simulink library "motohawk_engine_lib"  (Simulink 6.3)
undefined symbols (not defined in the file or in its folder): cast_val, IndPowerMax, InjSequence, lookup_group, MAF_Sensor_p, motohawk_tex, motohawk_vardec_config_group, motohawk_vardec_path, SampleTime, SparkSequence, SteadyStateECT, txtTitle, WarmUpTimeConst
libraries: MotoHawk_lib x234, motohawk_annotations_lib x22, motohawk_control_primitives_lib x20, motohawk_engine_lib x8, motohawk_control_primitives_lib_new x3
(part 6 of 7)

== system motohawk_engine_lib/Closed-Loop O2 Control - Single Bank/O2 Control State Determination ==
  note: Desired equivalence ratio is within a delta of 1.0 (stoichiometric)
  note: Engine indicated work is above a threshold.
      | Usually a few minutes of idle time, to allow sensor warm-up.
  note: There are no O2 sensor faults
  note: Closed-loop O2 control is disabled when running
      | enrichment or engine in ransient
  O2ControlEnable [bool] : Inport
  DesEquivRatio : Inport  Port=2
  IndWork [kJ] : Inport  Port=3
  O2 Sensor Fault : Inport  Port=4
  Constant : Constant  OutDataTypeMode=single
  Logical Operator : Logic  AllPortsSameDT=off
  Logical Operator1 : Logic  Inputs=5
  Logical Operator3 : Logic  Operator=NOT  Inputs=3
  Relational Operator : RelationalOperator  Operator=<=  ZeroCross=off  InputSameDT=on
  Relational Operator1 : RelationalOperator  ZeroCross=off  InputSameDT=on
  Relational Operator2 : RelationalOperator  ZeroCross=off  InputSameDT=on
  Sum : Sum  Inputs=|++  SaturateOnIntegerOverflow=on
  Sum1 : Sum  Inputs=+-|  SaturateOnIntegerOverflow=on
  motohawk_TitleBlock : motohawk_annotations_lib/motohawk_TitleBlock  BlockType_='Mototron_Title_Block'  ttl=[txtTitle '\newline\rmClosed-Loop O2 Control State Determination']  copyright="'THE INFORMATION CONTAINED IN THIS\\newlineDRAWING IS THE SOLE PROPERTY OF\\newlineMOTOTRON.  ANY REPRODUCTION IN\\newline PART OR AS A WHOLE WITHOUT THE\\newlineWRITTEN PERMISSION OF MOTOTRON\\newline IS PROHIBITED.\\fontsize{16}\\rm\\copyright\\rm\\fontsize{10} 2005'"  address='\fontsize{22}\it\fontname{Arial Black}MotoTron Corporation \fontname{Arial}\fontsize{10}\newline505 Marion Road, Oshkosh, WI, 54901\newlinewww.mototron.com (734) 822-7700'  image_file='mh.jpg'  pretty_print=on  edit_text=[motohawk_tex(get_param(bdroot, 'Description')) '\rm\newline' motohawk_tex(get_param(gcs, 'Name'))]  edit_as=6
  motohawk_calibration : MotoHawk_lib/Calibration & Probing Blocks/motohawk_calibration  nam='O2ReadyIndWork'  val=O2ReadyIndWork  storage=Calibration  show_more=on  name_source=Use Parameter  data_type=Inherit from 'Default Value'  read_level=1  write_level=1  ovr_cals=on  view_as=Number  enum_struct={'Disabled', 'Enabled'}  vector_style=Wide Row  use_help_units=on  help='Minimum indicated work from engine before closed-loop O2 control will be enabled'  units='kJ'  use_header_enum=off  row_header_enum={}  col_header_enum={}  use_min_max=on  min_val=0  max_val=inf  use_precision=off  precision=''  gain=1  offset=0  exp=1  use_mototune_group=on  mototune_group='Engine Control | Run | O2 Control | O2 Control Config'
  motohawk_calibration1 : MotoHawk_lib/Calibration & Probing Blocks/motohawk_calibration  nam='O2EquivRatioDelta'  val=O2EquivRatioDelta  storage=Calibration  show_more=on  name_source=Use Parameter  data_type=Inherit from 'Default Value'  read_level=1  write_level=1  ovr_cals=on  view_as=Number  enum_struct={'Disabled', 'Enabled'}  vector_style=Wide Row  use_help_units=on  help='Equivalence ratio must be within this delta of stoichiometric to allow closed-loop O2 control'  units='ratio'  use_header_enum=off  row_header_enum={}  col_header_enum={}  use_min_max=on  min_val=0  max_val=1.0  use_precision=off  precision=''  gain=1  offset=0  exp=1  use_mototune_group=on  mototune_group='Engine Control | Run | O2 Control | O2 Control Config'
  motohawk_calibration2 : MotoHawk_lib/Calibration & Probing Blocks/motohawk_calibration  nam='O2ControlEnable'  val=O2ControlEnable  storage=Calibration  show_more=on  name_source=Use Parameter  data_type=boolean  read_level=1  write_level=1  ovr_cals=on  view_as=Enumeration  enum_struct={'Disabled', 'Enabled'}  vector_style=Wide Row  use_help_units=on  help='When enabled, the closed-loop O2 control algorithm is used'  units=''  use_header_enum=off  row_header_enum={}  col_header_enum={}  use_min_max=off  min_val=-inf  max_val=inf  use_precision=off  precision=''  gain=1  offset=0  exp=1  use_mototune_group=on  mototune_group='Engine Control | Run | O2 Control | O2 Control Config'
  motohawk_probe : MotoHawk_lib/Calibration & Probing Blocks/motohawk_probe  nam='O2Control'  show_more=on  name_source=Use Parameter  read_level=1  view_as=Enumeration  enum_struct={'Open-Loop', 'Closed-Loop'}  vector_style=Wide Row  use_help_units=on  help='Indicates whether closed-loop O2 control is currently enabled'  units=''  use_header_enum=off  row_header_enum={}  col_header_enum={}  use_precision=off  precision=''  gain=1  offset=0  exp=1  use_mototune_group=on  mototune_group='Engine Control | Run | O2 Control'
  O2Control : Outport
  wires:
  Logical Operator3/1 -> Logical Operator1/4
  O2 Sensor Fault/1 -> Logical Operator3/1
  Logical Operator/1 -> Logical Operator1/3
  Relational Operator2/1 -> Logical Operator1/2
  motohawk_calibration/1 -> Relational Operator2/2
  IndWork [kJ]/1 -> Relational Operator2/1
  Relational Operator1/1 -> Logical Operator/2
  Relational Operator/1 -> Logical Operator/1
  Sum1/1 -> Relational Operator1/2
  Sum/1 -> Relational Operator/2
  DesEquivRatio/1 -> Relational Operator/1, Relational Operator1/1
  Constant/1 -> Sum1/1, Sum/2
  motohawk_calibration1/1 -> Sum1/2, Sum/1
  Logical Operator1/1 -> O2Control/1, motohawk_probe/1
  O2ControlEnable [bool]/1 -> Logical Operator1/1
  motohawk_calibration2/1 -> Logical Operator1/5

== system motohawk_engine_lib/Crank Synchronous SIgnal/Once at Startup ==
  note: Sample Signal Once at Startup
  Signal_Time : Inport
  f : TriggerPort  TriggerType=function-call
  Signal_StartUp : Outport
  wires:
  Signal_Time/1 -> Signal_StartUp/1

== system motohawk_engine_lib/Crank Synchronous SIgnal/TDC and MID_TDC ==
  note: Average of Signal on TDC and MID_TDC
  Signal_Time : Inport
  f : TriggerPort  TriggerType=function-call
  Gain : Gain  Gain=1/2  SaturateOnIntegerOverflow=on
  Sum : Sum  Inputs=|++  InputSameDT=on
  Unit Delay : UnitDelay  SampleTime=-1
  Signal_Ave : Outport
  wires:
  Signal_Time/1 -> Sum/1, Unit Delay/1
  Gain/1 -> Signal_Ave/1
  Sum/1 -> Gain/1
  Unit Delay/1 -> Sum/2

== system motohawk_engine_lib/Idle Governor/Idle State Determination ==
  note: Idle States
      | 1 - Flaring
      | 2 - OnIdle
      | 3 - OffIdle
  RPM : Inport
  TargetRPM : Inport  Port=2
  ThrPos [%] : Inport  Port=3
  Determine if RPM is Falling : Subsystem
  Idle State Machine : Stateflow chart
  OnIdle State : motohawk_control_primitives_lib/CompareTo  op===  val=2
  Relational Operator : RelationalOperator  Operator=<  ZeroCross=off  InputSameDT=on
  Relational Operator1 : RelationalOperator  Operator=<  ZeroCross=off  InputSameDT=on
  Relational Operator2 : RelationalOperator  ZeroCross=off  InputSameDT=on
  Sum : Sum  Inputs=|++  SaturateOnIntegerOverflow=on  InputSameDT=on
  motohawk_TitleBlock : motohawk_annotations_lib/motohawk_TitleBlock  BlockType_='Mototron_Title_Block'  ttl='Idle Governor State Determination'  copyright="'THE INFORMATION CONTAINED IN THIS\\newlineDRAWING IS THE SOLE PROPERTY OF\\newlineMOTOTRON.  ANY REPRODUCTION IN\\newline PART OR AS A WHOLE WITHOUT THE\\newlineWRITTEN PERMISSION OF MOTOTRON\\newline IS PROHIBITED.\\fontsize{16}\\rm\\copyright\\rm\\fontsize{10} 2005'"  address='\fontsize{22}\it\fontname{Arial Black}MotoTron Corporation \fontname{Arial}\fontsize{10}\newline505 Marion Road, Oshkosh, WI, 54901\newlinewww.mototron.com (734) 822-7700'  image_file='mh.jpg'  pretty_print=on  edit_text=[motohawk_tex(get_param(bdroot, 'Description')) '\rm\newline' motohawk_tex(get_param(gcs, 'Name'))]  edit_as=6
  motohawk_calibration1 : MotoHawk_lib/Calibration & Probing Blocks/motohawk_calibration  nam='IdleEntryRPMDelta'  val=200  storage=Calibration  show_more=on  name_source=Use Parameter  data_type=Inherit from 'Default Value'  read_level=1  write_level=1  ovr_cals=on  view_as=Number  enum_struct={'Disabled', 'Enabled'}  vector_style=Wide Row  use_help_units=on  help='RPM must be within this delta from IdleTargetRPM to enter the Idle governor'  units='RPM'  use_header_enum=off  row_header_enum={}  col_header_enum={}  use_min_max=off  min_val=-inf  max_val=inf  use_precision=off  precision=''  gain=1  offset=0  exp=1  use_mototune_group=off  mototune_group=motohawk_vardec_path(gcb)
  motohawk_calibration3 : MotoHawk_lib/Calibration & Probing Blocks/motohawk_calibration  nam='IdleEntryThrPosThresh'  val=10  storage=Calibration  show_more=on  name_source=Use Parameter  data_type=Inherit from 'Default Value'  read_level=1  write_level=1  ovr_cals=on  view_as=Number  enum_struct={'Disabled', 'Enabled'}  vector_style=Wide Row  use_help_units=on  help='The throttle position must be closed below this threshold to enter the Idle governor'  units='%'  use_header_enum=off  row_header_enum={}  col_header_enum={}  use_min_max=off  min_val=-inf  max_val=inf  use_precision=off  precision=''  gain=1  offset=0  exp=1  use_mototune_group=off  mototune_group=motohawk_vardec_path(gcb)
  motohawk_calibration4 : MotoHawk_lib/Calibration & Probing Blocks/motohawk_calibration  nam='IdleExitThrPosThresh'  val=15  storage=Calibration  show_more=on  name_source=Use Parameter  data_type=Inherit from 'Default Value'  read_level=1  write_level=1  ovr_cals=on  view_as=Number  enum_struct={'Disabled', 'Enabled'}  vector_style=Wide Row  use_help_units=on  help='The throttle position must be opened above this threshold to exit the Idle governor'  units='%'  use_header_enum=off  row_header_enum={}  col_header_enum={}  use_min_max=off  min_val=-inf  max_val=inf  use_precision=off  precision=''  gain=1  offset=0  exp=1  use_mototune_group=off  mototune_group=motohawk_vardec_path(gcb)
  motohawk_calibration6 : MotoHawk_lib/Calibration & Probing Blocks/motohawk_calibration  nam='IdleEnable'  val=true  storage=Display  show_more=on  name_source=Use Parameter  data_type=Inherit from 'Default Value'  read_level=1  write_level=1  ovr_cals=on  view_as=Number  enum_struct={'Disabled', 'Enabled'}  vector_style=Wide Row  use_help_units=on  help='Allows the Idle governor to be manually enabled and disabled'  units='bool'  use_header_enum=off  row_header_enum={}  col_header_enum={}  use_min_max=off  min_val=-inf  max_val=inf  use_precision=off  precision=''  gain=1  offset=0  exp=1  use_mototune_group=off  mototune_group=motohawk_vardec_path(gcb)
  motohawk_probe1 : MotoHawk_lib/Calibration & Probing Blocks/motohawk_probe  nam='IdleState'  show_more=on  name_source=Use Parameter  read_level=1  view_as=Number  enum_struct={'Disabled', 'Enabled'}  vector_style=Wide Row  use_help_units=on  help="'0 - Off Idle    1 - On Idle'"  units=''  use_header_enum=off  row_header_enum={}  col_header_enum={}  use_precision=off  precision=''  gain=1  offset=0  exp=1  use_mototune_group=off  mototune_group=motohawk_vardec_path(gcb)
  OnIdle : Outport
  wires:
  Relational Operator1/1 -> Idle State Machine/4(ThrPosLow)
  Relational Operator/1 -> Idle State Machine/3(RPMLow)
  OnIdle State/1 -> OnIdle/1
  Idle State Machine/1(IdleState) -> OnIdle State/1, motohawk_probe1/1
  motohawk_calibration6/1 -> Idle State Machine/1(IdleEnable)
  Relational Operator2/1 -> Idle State Machine/5(ThrPosHigh)
  motohawk_calibration4/1 -> Relational Operator2/2
  motohawk_calibration3/1 -> Relational Operator1/2
  Sum/1 -> Relational Operator/2
  motohawk_calibration1/1 -> Sum/1
  TargetRPM/1 -> Sum/2
  Determine if RPM is Falling/1(RPM Falling) -> Idle State Machine/2(RPMFalling)
  RPM/1 -> Determine if RPM is Falling/1(RPM), Relational Operator/1
  ThrPos [%]/1 -> Relational Operator2/1, Relational Operator1/1

== system motohawk_engine_lib/Idle Governor/Ramp RPM ==
  note: y[k] = a*x[k] + (1-a)*y[k-1]
  note: where a = t/T
  OnIdle : Inport
  RPM : Inport  Port=2
  TargetRPM : Inport  Port=3
  Constant : Constant
  Logical Operator : Logic  Operator=NOT
  Preload lowpass filter with current RPM while not on Idle : Switch  Threshold=1  ZeroCross=off  SaturateOnIntegerOverflow=on  InputSameDT=on
  Product1 : Product  Inputs=*/  SaturateOnIntegerOverflow=on  InputSameDT=on
  Product2 : Product  SaturateOnIntegerOverflow=on  InputSameDT=on
  Product3 : Product  SaturateOnIntegerOverflow=on  InputSameDT=on
  Sum : Sum  Inputs=-+|  SaturateOnIntegerOverflow=on
  Sum1 : Sum  SaturateOnIntegerOverflow=on
  Unit Delay : UnitDelay  Orientation=left  SampleTime=-1
  motohawk_TitleBlock : motohawk_annotations_lib/motohawk_TitleBlock  BlockType_='Mototron_Title_Block'  ttl='1st-Order Lowpass Filter\newlinewith Preload while not in Idle State'  copyright="'THE INFORMATION CONTAINED IN THIS\\newlineDRAWING IS THE SOLE PROPERTY OF\\newlineMOTOTRON.  ANY REPRODUCTION IN\\newline PART OR AS A WHOLE WITHOUT THE\\newlineWRITTEN PERMISSION OF MOTOTRON\\newline IS PROHIBITED.\\fontsize{16}\\rm\\copyright\\rm\\fontsize{10} 2005'"  address='\fontsize{22}\it\fontname{Arial Black}MotoTron Corporation \fontname{Arial}\fontsize{10}\newline505 Marion Road, Oshkosh, WI, 54901\newlinewww.mototron.com (734) 822-7700'  image_file='mh.jpg'  pretty_print=on  edit_text=[motohawk_tex(get_param(bdroot, 'Description')) '\rm\newline' motohawk_tex(get_param(gcs, 'Name'))]  edit_as=6
  motohawk_calibration : MotoHawk_lib/Calibration & Probing Blocks/motohawk_calibration  nam='IdleRPMRampFiltConst'  val=3  storage=Calibration  show_more=on  name_source=Use Parameter  data_type=Inherit from 'Default Value'  read_level=1  write_level=1  ovr_cals=on  view_as=Number  enum_struct={'Disabled', 'Enabled'}  vector_style=Wide Row  use_help_units=on  help='RPM ramp down time constant'  units='sec'  use_header_enum=off  row_header_enum={}  col_header_enum={}  use_min_max=off  min_val=-inf  max_val=inf  use_precision=off  precision=''  gain=1  offset=0  exp=1  use_mototune_group=on  mototune_group=motohawk_vardec_path(gcb)
  motohawk_delta_time : MotoHawk_lib/Extra Development Blocks/motohawk_delta_time  samp_time=SampleTime  init_val=0
  RPMSetPt : Outport
  wires:
  RPM/1 -> Preload lowpass filter with current RPM while not on Idle/1
  TargetRPM/1 -> Product2/1
  Logical Operator/1 -> Preload lowpass filter with current RPM while not on Idle/2
  Product1/1 -> Sum/1, Product2/2  "alpha"
  Constant/1 -> Sum/2
  Product2/1 -> Sum1/1
  Product3/1 -> Sum1/2
  Sum/1 -> Product3/1
  Unit Delay/1 -> Product3/2
  motohawk_delta_time/1 -> Product1/1
  motohawk_calibration/1 -> Product1/2
  Sum1/1 -> Preload lowpass filter with current RPM while not on Idle/3
  Preload lowpass filter with current RPM while not on Idle/1 -> Unit Delay/1, RPMSetPt/1
  OnIdle/1 -> Logical Operator/1

== system motohawk_engine_lib/Linear Sensor Characterization/If Action Subsystem ==
  In : Inport
  Action Port : ActionPort
  Out : Outport
  wires:
  In/1 -> Out/1

== system motohawk_engine_lib/Linear Sensor Characterization/If Action Subsystem1 ==
  In : Inport
  Action Port : ActionPort
  Out : Outport
  wires:
  In/1 -> Out/1

== system motohawk_engine_lib/Linear Sensor Characterization/If Action Subsystem2 ==
  In : Inport
  Action Port : ActionPort
  Out : Outport
  wires:
  In/1 -> Out/1

== system motohawk_engine_lib/Linear Sensor Characterization w Adapt/ADAPT SCALING ==
  MIN_MAX : Inport
  ADAPT_LIMTS : Inport  Port=2
  ADAPT_LO_REQUEST : Inport  Port=3
  ADAPT_HI_REQUEST : Inport  Port=4
  ADAPT HI : Subsystem
  ADAPT LO : Subsystem
  Bus Selector : BusSelector  OutputSignals=adapt_lo_max,adapt_lo_min
  Bus Selector1 : BusSelector  OutputSignals=adapt_hi_max,adapt_hi_min
  Bus Selector2 : BusSelector  OutputSignals=max_last5,min_last5
  MinMax : MinMax  Inputs=2
  MinMax1 : MinMax  Function=max  Inputs=2
  MinMaxFilter : Subsystem
  motohawk_calibration1 : MotoHawk_lib/Calibration & Probing Blocks/motohawk_calibration  nam=[prefix 'AdaptLoEnable']  val=true  storage=Calibration  show_more=on  name_source=Use Parameter  data_type=Inherit from 'Default Value'  read_level=1  write_level=1  ovr_cals=on  view_as=Enumeration  enum_struct={'Disabled', 'Enabled'}  vector_style=Wide Row  use_help_units=on  help='Enables or disables this adapt.'  units=''  use_header_enum=off  row_header_enum={}  col_header_enum={}  use_min_max=off  min_val=-inf  max_val=inf  use_precision=off  precision=''  gain=1  offset=0  exp=1  use_mototune_group=on  mototune_group=[group ' | ' nam ' Config']
  motohawk_calibration14 : MotoHawk_lib/Calibration & Probing Blocks/motohawk_calibration  nam=[prefix 'Adapt_Delta']  val=5  storage=Calibration  show_more=on  name_source=Use Parameter  data_type=Inherit from 'Default Value'  read_level=1  write_level=1  ovr_cals=on  view_as=Number  enum_struct={'Disabled', 'Enabled'}  vector_style=Wide Row  use_help_units=on  help='Specifies the minimum deviation amount to react to.'  units='ADC'  use_header_enum=off  row_header_enum={}  col_header_enum={}  use_min_max=off  min_val=-inf  max_val=inf  use_precision=off  precision=''  gain=1  offset=0  exp=1  use_mototune_group=on  mototune_group=[group ' | ' nam ' Config']
  motohawk_calibration2 : MotoHawk_lib/Calibration & Probing Blocks/motohawk_calibration  nam=[prefix 'AdaptHiEnable']  val=true  storage=Calibration  show_more=on  name_source=Use Parameter  data_type=Inherit from 'Default Value'  read_level=1  write_level=1  ovr_cals=on  view_as=Enumeration  enum_struct={'Disabled', 'Enabled'}  vector_style=Wide Row  use_help_units=on  help='Enables or disables this adapt.'  units=''  use_header_enum=off  row_header_enum={}  col_header_enum={}  use_min_max=off  min_val=-inf  max_val=inf  use_precision=off  precision=''  gain=1  offset=0  exp=1  use_mototune_group=on  mototune_group=[group ' | ' nam ' Config']
  motohawk_data_read : MotoHawk_lib/Data Storage Blocks/motohawk_data_read  source=Lookup By Name  structure=Scalar  operation=Read entire data structure at once  sz_vec=4  sz_row=2  sz_col=3  typ=uint16  nam=[prefix 'Raw_Adpt_Low']  checkNull=on  struct_inst_name='Struct1'
  motohawk_data_read1 : MotoHawk_lib/Data Storage Blocks/motohawk_data_read  source=Lookup By Name  structure=Scalar  operation=Read entire data structure at once  sz_vec=4  sz_row=2  sz_col=3  typ=uint16  nam=[prefix 'Raw_Adpt_Hi']  checkNull=on  struct_inst_name='Struct1'
  ADAPTED_HI_ENDPT : Outport
  ADAPTED_LO_ENDPT : Outport  Port=2
  wires:
  ADAPT_HI_REQUEST/1 -> ADAPT HI/1(ADAPT_REQUEST)
  motohawk_calibration2/1 -> ADAPT HI/2(ADAPT_ENABLE)
  ADAPT_LO_REQUEST/1 -> ADAPT LO/1(ADAPT_REQUEST)
  motohawk_calibration1/1 -> ADAPT LO/2(ADAPT_ENABLE)
  motohawk_data_read1/1 -> MinMax1/1
  MinMax1/1 -> ADAPT HI/3(CUR_ADAPT_PT)
  motohawk_data_read/1 -> MinMax/1
  MinMax/1 -> ADAPT LO/3(CUR_ADAPT_PT)
  ADAPT_LIMTS/1 -> Bus Selector/1, Bus Selector1/1
  Bus Selector/1 -> MinMax/2, ADAPT LO/4(ADAPT_RANGE_MAX)  "<adapt_lo_max>"
  Bus Selector/2 -> ADAPT LO/5(ADAPT_RANGE_MIN)  "<adapt_lo_min>"
  motohawk_calibration14/1 -> ADAPT HI/6(ADAPT_MIN_DELTA), ADAPT LO/6(ADAPT_MIN_DELTA)
  ADAPT LO/1(ADAPTED_ENDPT) -> ADAPTED_LO_ENDPT/1
  ADAPT HI/1(ADAPTED_ENDPT) -> ADAPTED_HI_ENDPT/1
  Bus Selector1/1 -> ADAPT HI/4(ADAPT_RANGE_MAX)  "<adapt_hi_max>"
  Bus Selector1/2 -> ADAPT HI/5(ADAPT_RANGE_MIN), MinMax1/2  "<adapt_hi_min>"
  MIN_MAX/1 -> MinMaxFilter/1(Input)
  Bus Selector2/1 -> ADAPT LO/7(MAX_LAST5)  "<max_last5>"
  Bus Selector2/2 -> ADAPT HI/7(MAX_LAST5)  "<min_last5>"
  MinMaxFilter/1(Min_Max) -> Bus Selector2/1

== system motohawk_engine_lib/Linear Sensor Characterization w Adapt/FAULTS ==
  INPUT_FILT : Inport
  ADAPT_PT_HI : Inport  Port=2
  ADAPT_PT_LO : Inport  Port=3
  ADAPT_LIMTS : Inport  Port=4
  Bus Selector : BusSelector  OutputSignals=adapt_lo_max,adapt_lo_min,adapt_hi_max,adapt_hi_min
  Relational Operator : RelationalOperator  Operator=>
  Relational Operator1 : RelationalOperator  Operator=<
  Relational Operator2 : RelationalOperator  Operator=<
  Relational Operator3 : RelationalOperator  Operator=>
  Relational Operator4 : RelationalOperator  Operator=<
  Relational Operator5 : RelationalOperator  Operator=>
  motohawk_calibration5 : MotoHawk_lib/Calibration & Probing Blocks/motohawk_calibration  nam=[prefix 'InputHiFltPos']  val=1020  storage=Calibration  show_more=on  name_source=Use Parameter  data_type=Inherit from 'Default Value'  read_level=1  write_level=1  ovr_cals=on  view_as=Number  enum_struct={'Disabled', 'Enabled'}  vector_style=Wide Row  use_help_units=on  help='Hi limit of input signal which sets fault'  units='ADC'  use_header_enum=off  row_header_enum={}  col_header_enum={}  use_min_max=off  min_val=-inf  max_val=inf  use_precision=off  precision=''  gain=1  offset=0  exp=1  use_mototune_group=on  mototune_group=[group ' | ' nam ' Config']
  motohawk_calibration6 : MotoHawk_lib/Calibration & Probing Blocks/motohawk_calibration  nam=[prefix 'InputLoFltPos']  val=10  storage=Calibration  show_more=on  name_source=Use Parameter  data_type=Inherit from 'Default Value'  read_level=1  write_level=1  ovr_cals=on  view_as=Number  enum_struct={'Disabled', 'Enabled'}  vector_style=Wide Row  use_help_units=on  help='Low limit of input signal which sets fault'  units='ADC'  use_header_enum=off  row_header_enum={}  col_header_enum={}  use_min_max=off  min_val=-inf  max_val=inf  use_precision=off  precision=''  gain=1  offset=0  exp=1  use_mototune_group=on  mototune_group=[group ' | ' nam ' Config']
  motohawk_fault_def1 : MotoHawk_lib/Fault Management Blocks/motohawk_fault_def  nam=[prefix 'AdaptLoMax']  mode=Enabled  id=[]  x=25  y=50  input_suspected=on  indeterminate=off  increment_xy=on  downsample_count=1  ovr_cals=on  ovr_actions=on  show_actions=off  action1_name=''  action1_cond=(None)  action2_name=''  action2_cond=(None)  action3_name=''  action3_cond=(None)  action4_name=''  action4_cond=(None)
  motohawk_fault_def2 : MotoHawk_lib/Fault Management Blocks/motohawk_fault_def  nam=[prefix 'AdaptHiMax']  mode=Enabled  id=[]  x=25  y=50  input_suspected=on  indeterminate=off  increment_xy=on  downsample_count=1  ovr_cals=on  ovr_actions=on  show_actions=off  action1_name=''  action1_cond=(None)  action2_name=''  action2_cond=(None)  action3_name=''  action3_cond=(None)  action4_name=''  action4_cond=(None)
  motohawk_fault_def3 : MotoHawk_lib/Fault Management Blocks/motohawk_fault_def  nam=[prefix 'AdaptHiMin']  mode=Enabled  id=[]  x=25  y=50  input_suspected=on  indeterminate=off  increment_xy=on  downsample_count=1  ovr_cals=on  ovr_actions=on  show_actions=off  action1_name=''  action1_cond=(None)  action2_name=''  action2_cond=(None)  action3_name=''  action3_cond=(None)  action4_name=''  action4_cond=(None)
  motohawk_fault_def4 : MotoHawk_lib/Fault Management Blocks/motohawk_fault_def  nam=[prefix 'RangeHigh']  mode=Enabled  id=[]  x=25  y=50  input_suspected=on  indeterminate=off  increment_xy=on  downsample_count=1  ovr_cals=on  ovr_actions=on  show_actions=off  action1_name=''  action1_cond=(None)  action2_name=''  action2_cond=(None)  action3_name=''  action3_cond=(None)  action4_name=''  action4_cond=(None)
  motohawk_fault_def5 : MotoHawk_lib/Fault Management Blocks/motohawk_fault_def  nam=[prefix 'RangeLow']  mode=Enabled  id=[]  x=25  y=50  input_suspected=on  indeterminate=off  increment_xy=on  downsample_count=1  ovr_cals=on  ovr_actions=on  show_actions=off  action1_name=''  action1_cond=(None)  action2_name=''  action2_cond=(None)  action3_name=''  action3_cond=(None)  action4_name=''  action4_cond=(None)
  motohawk_fault_def8 : MotoHawk_lib/Fault Management Blocks/motohawk_fault_def  nam=[prefix 'AdaptLoMin']  mode=Enabled  id=[]  x=25  y=50  input_suspected=on  indeterminate=off  increment_xy=on  downsample_count=1  ovr_cals=on  ovr_actions=on  show_actions=off  action1_name=''  action1_cond=(None)  action2_name=''  action2_cond=(None)  action3_name=''  action3_cond=(None)  action4_name=''  action4_cond=(None)
  wires:
  ADAPT_LIMTS/1 -> Bus Selector/1
  Bus Selector/1 -> Relational Operator/2  "<adapt_lo_max>"
  Bus Selector/2 -> Relational Operator1/2  "<adapt_lo_min>"
  Bus Selector/3 -> Relational Operator3/2  "<adapt_hi_max>"
  Bus Selector/4 -> Relational Operator2/2  "<adapt_hi_min>"
  ADAPT_PT_LO/1 -> Relational Operator/1, Relational Operator1/1
  ADAPT_PT_HI/1 -> Relational Operator2/1, Relational Operator3/1
  INPUT_FILT/1 -> Relational Operator4/1, Relational Operator5/1
  motohawk_calibration6/1 -> Relational Operator4/2
  motohawk_calibration5/1 -> Relational Operator5/2
  Relational Operator4/1 -> motohawk_fault_def5/1
  Relational Operator5/1 -> motohawk_fault_def4/1
  Relational Operator/1 -> motohawk_fault_def1/1
  Relational Operator1/1 -> motohawk_fault_def8/1
  Relational Operator3/1 -> motohawk_fault_def2/1
  Relational Operator2/1 -> motohawk_fault_def3/1

== system motohawk_engine_lib/Linear Sensor Characterization w Adapt/SENSOR FAULT MANAGER ==
  Signal : Inport
  Default : Inport  Port=2
  If : If  Orientation=down  NumInputs=2  IfExpression=u1  ElseIfExpressions=u2  ZeroCross=off
  If Action Subsystem : motohawk_engine_lib/Linear Sensor Characterization/If Action Subsystem
  If Action Subsystem1 : motohawk_engine_lib/Linear Sensor Characterization/If Action Subsystem1
  If Action Subsystem2 : motohawk_engine_lib/Linear Sensor Characterization/If Action Subsystem2
  Logical Operator1 : Logic  Operator=OR
  Logical Operator4 : Logic  Operator=OR
  Logical Operator5 : Logic
  Logical Operator6 : Logic  Operator=NOT
  Merge : Merge  Inputs=3
  Override : MotoHawk_lib/Calibration & Probing Blocks/motohawk_override_abs  parent_name=nam  show_more=on  name_source=Use Parameter  parent_read_level=1  parent_override_level=1  view_as=Number  enum_struct={'Disabled', 'Enabled'}  use_help_units=on  parent_help='Override result of linear sensor characterization, in engineering units'  parent_units=units  use_min_max=on  parent_min=-inf  parent_max=inf  use_precision=off  parent_precision=''  parent_gain=1  parent_offset=0  parent_exp=1  use_mototune_group=on  parent_group=group
  Unit Delay1 : UnitDelay  Orientation=left  SampleTime=-1
  motohawk_fault_status1 : MotoHawk_lib/Fault Management Blocks/motohawk_fault_status  source=Lookup By Name  nam=[prefix 'RangeHigh']  status=Active
  motohawk_fault_status2 : MotoHawk_lib/Fault Management Blocks/motohawk_fault_status  source=Lookup By Name  nam=[prefix 'RangeHigh']  status=Suspected
  motohawk_fault_status3 : MotoHawk_lib/Fault Management Blocks/motohawk_fault_status  source=Lookup By Name  nam=[prefix 'RangeLow']  status=Suspected
  motohawk_fault_status4 : MotoHawk_lib/Fault Management Blocks/motohawk_fault_status  source=Lookup By Name  nam=[prefix 'RangeLow']  status=Active
  Out : Outport
  wires:
  Merge/1 -> Override/1, Unit Delay1/1
  If/3 -> If Action Subsystem2/Action
  If/1 -> If Action Subsystem/Action
  If Action Subsystem2/1 -> Merge/1
  If Action Subsystem/1 -> Merge/2
  Signal/1 -> If Action Subsystem2/1
  If Action Subsystem1/1 -> Merge/3
  If/2 -> If Action Subsystem1/Action
  Unit Delay1/1 -> If Action Subsystem/1
  Default/1 -> If Action Subsystem1/1
  Override/1 -> Out/1
  motohawk_fault_status2/1 -> Logical Operator1/1
  motohawk_fault_status3/1 -> Logical Operator1/2
  motohawk_fault_status1/1 -> Logical Operator4/1
  motohawk_fault_status4/1 -> Logical Operator4/2
  Logical Operator6/1 -> Logical Operator5/1
  Logical Operator5/1 -> If/1
  Logical Operator1/1 -> Logical Operator5/2
  Logical Operator4/1 -> Logical Operator6/1, If/2

== system motohawk_engine_lib/Load, Torque, Power, Work - Using APC/Calculate Power and Work ==
  IndTorque (N*m) : Inport
  RPM : Inport  Port=2
  Data Type Conversion : DataTypeConversion  SaturateOnIntegerOverflow=on  RndMeth=Zero
  Ground : Ground
  Integrate Power to Compute Work : motohawk_control_primitives_lib/Integrator  samp_time=SampleTime
  Mux1 : Mux  Inputs=2
  Torque to Power : Fcn  Expr=u(1)*u(2)*pi/30000
  motohawk_TitleBlock : motohawk_annotations_lib/motohawk_TitleBlock  BlockType_='Mototron_Title_Block'  ttl='Calculate Observed Engine States, such as Load, Torque, and Power\newline\rmUsing Airflow rate, calculate Air per Cylinder, and lookup Load and Torque values.'  copyright="'THE INFORMATION CONTAINED IN THIS\\newlineDRAWING IS THE SOLE PROPERTY OF\\newlineMOTOTRON.  ANY REPRODUCTION IN\\newline PART OR AS A WHOLE WITHOUT THE\\newlineWRITTEN PERMISSION OF MOTOTRON\\newline IS PROHIBITED.\\fontsize{16}\\rm\\copyright\\rm\\fontsize{10} 2005'"  address='\fontsize{22}\it\fontname{Arial Black}MotoTron Corporation \fontname{Arial}\fontsize{10}\newline505 Marion Road, Oshkosh, WI, 54901\newlinewww.mototron.com (734) 822-7700'  image_file='mh.jpg'  pretty_print=on  edit_text=[motohawk_tex(get_param(bdroot, 'Description')) '\rm\newline' motohawk_tex(get_param(gcs, 'Name'))]  edit_as=6
  motohawk_calibration : MotoHawk_lib/Calibration & Probing Blocks/motohawk_calibration  nam='IndWorkMax'  val=inf  storage=Calibration  show_more=on  name_source=Use Parameter  data_type=Inherit from 'Default Value'  read_level=1  write_level=1  ovr_cals=on  view_as=Number  enum_struct={'Disabled', 'Enabled'}  vector_style=Wide Row  use_help_units=on  help='Maximum Indicated Work'  units='kJ'  use_header_enum=off  row_header_enum={}  col_header_enum={}  use_min_max=off  min_val=-inf  max_val=inf  use_precision=off  precision=''  gain=1  offset=0  exp=1  use_mototune_group=on  mototune_group=lookup_group(gcb)
  motohawk_probe : MotoHawk_lib/Calibration & Probing Blocks/motohawk_probe  nam='IndPower'  show_more=on  name_source=Use Parameter  read_level=1  view_as=Number  enum_struct={'Disabled', 'Enabled'}  vector_style=Wide Row  use_help_units=on  help='Indicated Power'  units='kW'  use_header_enum=off  row_header_enum={}  col_header_enum={}  use_precision=off  precision=''  gain=1  offset=0  exp=1  use_mototune_group=on  mototune_group=lookup_group(gcb)
  motohawk_probe1 : MotoHawk_lib/Calibration & Probing Blocks/motohawk_probe  nam='IndWork'  show_more=on  name_source=Use Parameter  read_level=1  view_as=Number  enum_struct={'Disabled', 'Enabled'}  vector_style=Wide Row  use_help_units=on  help='Indicated Work'  units='kJ'  use_header_enum=off  row_header_enum={}  col_header_enum={}  use_precision=off  precision=''  gain=1  offset=0  exp=1  use_mototune_group=on  mototune_group=lookup_group(gcb)
  IndPower (kW) : Outport
  IndWork (kJ) : Outport  Port=2
  wires:
  Mux1/1 -> Data Type Conversion/1
  Data Type Conversion/1 -> Torque to Power/1
  Torque to Power/1 -> Integrate Power to Compute Work/1, IndPower (kW)/1, motohawk_probe/1
  Integrate Power to Compute Work/1 -> IndWork (kJ)/1, motohawk_probe1/1
  motohawk_calibration/1 -> Integrate Power to Compute Work/5
  IndTorque (N*m)/1 -> Mux1/1
  RPM/1 -> Mux1/2
  Ground/1 -> Integrate Power to Compute Work/3, Integrate Power to Compute Work/2, Integrate Power to Compute Work/4

== system motohawk_engine_lib/Mass Flow to Charge Mass Transform/Multiply and Divide, avoiding divde by zero ==
  X1 : Inport
  "X2 " : Inport  Port=2
  Divide1 : Inport  Port=3
  Divide2 : Inport  Port=4
  Enable : EnablePort  StatesWhenEnabling=reset
  charge mass : Product  Inputs=**//  SaturateOnIntegerOverflow=on  InputSameDT=on
  " " : Outport
  wires:
  charge mass/1 -> " "/1
  "X2 "/1 -> charge mass/2
  X1/1 -> charge mass/1
  Divide1/1 -> charge mass/3
  Divide2/1 -> charge mass/4

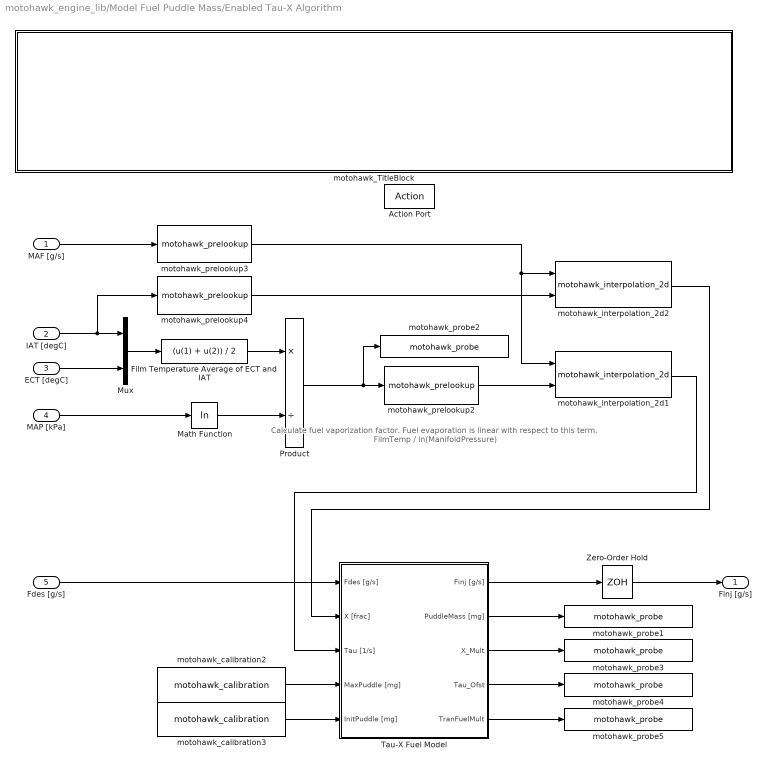
== system motohawk_engine_lib/Model Fuel Puddle Mass/Enabled Tau-X Algorithm ==
  note: Calculate fuel vaporization factor.
      | Fuel evaporation is linear with respect to this term.
      | FilmTemp / ln(ManifoldPressure)
  MAF [g/s] : Inport
  IAT [degC] : Inport  Port=2
  ECT [degC] : Inport  Port=3
  MAP [kPa] : Inport  Port=4
  Fdes [g/s] : Inport  Port=5
  Action Port : ActionPort  InitializeStates=reset
  Film Temperature Average of ECT and IAT : Fcn  Expr=(u(1) + u(2)) / 2
  Math Function : Math  Operator=log  SaturateOnIntegerOverflow=on
  Mux : Mux  Inputs=2
  Product : Product  Inputs=*/  SaturateOnIntegerOverflow=on  InputSameDT=on
  Tau-X Fuel Model : Subsystem  mask{samp_time=SampleTime}
      mask prompts: samp_time "Sample Time"
      mask Display:
      | patch([0 0 1 1], 0.5*[0 0.075 0.075 0], [230/255 0/255 0/255])
      | patch([0 0 1 1], 0.5*[0.025 0.05 0.05 0.025], [150/255 0/255 0/255])
      | patch([0 0 1 1], 0.5*[0 0.025 0.025 0], [0/255 0/255 0/255])
      | 
      | disp('TRANSIENT FUELING\nTAU-X MODEL');
  Zero-Order Hold : ZeroOrderHold  SampleTime=-1
  motohawk_TitleBlock : Subsystem  mask{BlockType_='Mototron_Title_Block', ttl=[txtTitle '\newline\rmPer-Cylinder Transient Fueling Model\newlineSchedule Tau and X parameters on RPM and load'], im=mh.jpg}
      mask prompts: ttl "Description"; im "Image FIle"
      mask init:
      | set_param(gcb,'BlockType_','''Mototron_Title_Block''')
      | set_param(gcb,'MaskVisibilityString','off,on,on');
      mask Display:
      | image(imread(im),[0.31 0.66 0.31 0.35])
      | 
      | plot([0 0 1 1 0],[0 1 1 0 0])
      | plot([.3 1],[0.65 0.65])
      | plot([.3 .3],[0.1 1.0])
      | plot([0 1],[0.1 0.1])
      | plot([0.91 0.91],[0 0.1])
      | text(1,1,'\fontsize{22}\it\fontname{Arial Black}MotoTron Corporation \fontname{Arial}\fontsize{10}\newline505 Marion Road, Oshkosh, WI, 54901\newlinewww.mototron.com (734) 822-7700','verticalAlignment','Top','horizontalAlignment','Right','texmode','on')
      | text(0.01,1,['\fontsize{14}\it\bfPROPRIETARY\newlineAND CONFIDENTIAL\newline\fontsize{10}
      | THE INFORMATION CONTAINED IN THIS\newline
      | DRAWING IS THE SOLE PROPERTY OF\newline
      | MOTOTRON.  ANY REPRODUCTION IN\newline
      | PART OR AS A WHOLE WITHOUT THE\newline
      | WRITTEN PERMISSION OF MOTOTRON\newline
      | IS PROHIBITED.\fontsize{16}\rm\copyright\rm\fontsize{10} 2004' ],'verticalAlignment','Top','horizontalAlignment','Left','texmode','on')
      | 
      | text(0.9,0,['\fontsize{11}\bfPath: \rm' strrep(motohawk_vardec_path(gcb),'_','\_')],'verticalAlignment','Bottom','horizontalAlignment','Right','texmode','on')
      | text(0.31,0.65,['\fontsize{10}\bfDescription:'],'verticalAlignment','Top','horizontalAlignment','Left','texmode','on')
      | 
      | text(0.31,0.55,['\fontsize{14}\bf' ttl],'verticalAlignment','Top','horizontalAlignment','Left','texmode','on')
      | text(0.99,0,['\fontsize{11}\bfREV: \rm' motohawk_build_version],'verticalAlignment','Bottom','horizontalAlignment','Right','texmode','on')
  motohawk_calibration2 : MotoHawk_lib/Calibration & Probing Blocks/motohawk_calibration  nam='TransientFuelMaxPuddle'  val=0  storage=Calibration  show_more=on  name_source=Use Parameter  data_type=Inherit from 'Default Value'  read_level=1  write_level=1  ovr_cals=on  view_as=Number  enum_struct={'Disabled', 'Enabled'}  vector_style=Wide Row  use_help_units=on  help='Maximum fuel puddle size'  units='mg'  use_header_enum=off  row_header_enum={}  col_header_enum={}  use_min_max=on  min_val=0  max_val=inf  use_precision=off  precision=''  gain=1  offset=0  exp=1  use_mototune_group=on  mototune_group=group_cal
  motohawk_calibration3 : MotoHawk_lib/Calibration & Probing Blocks/motohawk_calibration  nam='TransientFuelInitPuddle'  val=0  storage=Calibration  show_more=on  name_source=Use Parameter  data_type=Inherit from 'Default Value'  read_level=1  write_level=1  ovr_cals=on  view_as=Number  enum_struct={'Disabled', 'Enabled'}  vector_style=Wide Row  use_help_units=on  help='Initial fuel puddle size'  units='mg'  use_header_enum=off  row_header_enum={}  col_header_enum={}  use_min_max=on  min_val=0  max_val=inf  use_precision=off  precision=''  gain=1  offset=0  exp=1  use_mototune_group=on  mototune_group=group_cal
  motohawk_interpolation_2d1 : MotoHawk_lib/Lookup Tables/motohawk_interpolation_2d  nam='TransientFuelTau'  table_data=ones(5,5)  show_more=on  data_type=Inherit from 'Table Data'  storage=NonAdaptive  read_level=1  write_level=1  ovr_cals=on  use_help=on  help='Fuel evaporation time constant'  units='sec'  use_min_max=on  min_val=SampleTime  max_val=inf  use_precision=off  precision=''  gain=1  offset=0  exp=1  use_links=off  row_prelookup_block=''  col_prelookup_block=''  output_name=''  use_mototune_group=on  mototune_group=group_cal
  motohawk_interpolation_2d2 : MotoHawk_lib/Lookup Tables/motohawk_interpolation_2d  nam='TransientFuelX'  table_data=ones(5,5)  show_more=on  data_type=Inherit from 'Table Data'  storage=NonAdaptive  read_level=1  write_level=1  ovr_cals=on  use_help=on  help='Fraction of injected fuel to enter the puddle'  units='frac'  use_min_max=on  min_val=0  max_val=1  use_precision=off  precision=''  gain=1  offset=0  exp=1  use_links=off  row_prelookup_block=''  col_prelookup_block=''  output_name=''  use_mototune_group=on  mototune_group=group_cal
  motohawk_prelookup2 : MotoHawk_lib/Lookup Tables/motohawk_prelookup  nam='FuelVapFactor'  breakpoint_data=ones(1,5)  show_more=on  data_type=Inherit from 'Table Data'  storage=Constant  read_level=1  write_level=1  ovr_cals=on  use_help=on  help='Breakpoints for fuel vaporization factor'  units='degC/log(kPa)'  use_min_max=off  min_val=-inf  max_val=inf  use_precision=off  precision=''  gain=1  offset=0  exp=1  use_links=on  input_name=''  use_mototune_group=on  mototune_group='Indexes'
  motohawk_prelookup3 : MotoHawk_lib/Lookup Tables/motohawk_prelookup  nam='MAF05'  breakpoint_data=ones(1,5)  show_more=on  data_type=Inherit from 'Table Data'  storage=Constant  read_level=1  write_level=1  ovr_cals=on  use_help=on  help='Breakpoints for Mass Airflow'  units='g/s'  use_min_max=off  min_val=-inf  max_val=inf  use_precision=off  precision=''  gain=1  offset=0  exp=1  use_links=on  input_name='MAF'  use_mototune_group=on  mototune_group='Indexes'
  motohawk_prelookup4 : MotoHawk_lib/Lookup Tables/motohawk_prelookup  nam='IAT05'  breakpoint_data=ones(1,5)  show_more=on  data_type=Inherit from 'Table Data'  storage=Constant  read_level=1  write_level=1  ovr_cals=on  use_help=on  help='Breakpoints for intake air temperature'  units='degC'  use_min_max=off  min_val=-inf  max_val=inf  use_precision=off  precision=''  gain=1  offset=0  exp=1  use_links=on  input_name='IAT'  use_mototune_group=on  mototune_group='Indexes'
  motohawk_probe1 : MotoHawk_lib/Calibration & Probing Blocks/motohawk_probe  nam='TransientFuelPuddleMass'  show_more=on  name_source=Use Parameter  read_level=1  view_as=Number  enum_struct={'Disabled', 'Enabled'}  vector_style=Wide Row  use_help_units=on  help='Current modeled fuel puddle mass for Tau-X transient fuel'  units='mg'  use_header_enum=off  row_header_enum={}  col_header_enum={}  use_precision=off  precision=''  gain=1  offset=0  exp=1  use_mototune_group=on  mototune_group=group_dis
  motohawk_probe2 : MotoHawk_lib/Calibration & Probing Blocks/motohawk_probe  nam='FuelVapFactor'  show_more=on  name_source=Use Parameter  read_level=1  view_as=Number  enum_struct={'Disabled', 'Enabled'}  vector_style=Wide Row  use_help_units=on  help='Fuel vaporization factor - Fuel evaporation is linear with respect to this term'  units='degC/log(kPa)'  use_header_enum=off  row_header_enum={}  col_header_enum={}  use_precision=off  precision=''  gain=1  offset=0  exp=1  use_mototune_group=on  mototune_group=group_dis
  motohawk_probe3 : MotoHawk_lib/Calibration & Probing Blocks/motohawk_probe  nam='TransientFuel_X_Mult'  show_more=on  name_source=Use Parameter  read_level=1  view_as=Number  enum_struct={'Disabled', 'Enabled'}  vector_style=Wide Row  use_help_units=on  help='Multiplier on desired fuel flow due to X contribution (1/(1-X)).'  units=''  use_header_enum=off  row_header_enum={}  col_header_enum={}  use_precision=off  precision=''  gain=1  offset=0  exp=1  use_mototune_group=on  mototune_group=group_dis
  motohawk_probe4 : MotoHawk_lib/Calibration & Probing Blocks/motohawk_probe  nam='TransientFuel_Tau_Ofst'  show_more=on  name_source=Use Parameter  read_level=1  view_as=Number  enum_struct={'Disabled', 'Enabled'}  vector_style=Wide Row  use_help_units=on  help='Offset applied to desired fuel flow based on Tau contribution (-M_pud/Tau).'  units='g/s'  use_header_enum=off  row_header_enum={}  col_header_enum={}  use_precision=off  precision=''  gain=1  offset=0  exp=1  use_mototune_group=on  mototune_group=group_dis
  motohawk_probe5 : MotoHawk_lib/Calibration & Probing Blocks/motohawk_probe  nam='TransientFuel_Total_Mult'  show_more=on  name_source=Use Parameter  read_level=1  view_as=Number  enum_struct={'Disabled', 'Enabled'}  vector_style=Wide Row  use_help_units=on  help='Total transient fuel multiplier applied to desired fuel flow resulting from Tau-X model.'  units=''  use_header_enum=off  row_header_enum={}  col_header_enum={}  use_precision=off  precision=''  gain=1  offset=0  exp=1  use_mototune_group=on  mototune_group=group_dis
  Finj [g/s] : Outport
  wires:
  Tau-X Fuel Model/5(TranFuelMult) -> motohawk_probe5/1
  Tau-X Fuel Model/4(Tau_Ofst) -> motohawk_probe4/1
  Tau-X Fuel Model/3(X_Mult) -> motohawk_probe3/1
  motohawk_calibration2/1 -> Tau-X Fuel Model/4(MaxPuddle [mg])
  motohawk_calibration3/1 -> Tau-X Fuel Model/5(InitPuddle [mg])
  Tau-X Fuel Model/2(PuddleMass [mg]) -> motohawk_probe1/1
  Mux/1 -> Film Temperature Average of ECT and IAT/1
  Film Temperature Average of ECT and IAT/1 -> Product/1
  Math Function/1 -> Product/2
  Product/1 -> motohawk_prelookup2/1, motohawk_probe2/1
  IAT [degC]/1 -> Mux/1, motohawk_prelookup4/1
  motohawk_prelookup3/1 -> motohawk_interpolation_2d2/1, motohawk_interpolation_2d1/1
  motohawk_prelookup4/1 -> motohawk_interpolation_2d2/2
  Fdes [g/s]/1 -> Tau-X Fuel Model/1(Fdes [g/s])
  MAF [g/s]/1 -> motohawk_prelookup3/1
  ECT [degC]/1 -> Mux/2
  MAP [kPa]/1 -> Math Function/1
  Tau-X Fuel Model/1(Finj [g/s]) -> Zero-Order Hold/1
  Zero-Order Hold/1 -> Finj [g/s]/1
  motohawk_prelookup2/1 -> motohawk_interpolation_2d1/2
  motohawk_interpolation_2d1/1 -> Tau-X Fuel Model/3(Tau [1/s])
  motohawk_interpolation_2d2/1 -> Tau-X Fuel Model/2(X [frac])

== system motohawk_engine_lib/Model Fuel Puddle Mass/Pass-Through ==
  note: Simply pass-through desired fuel as injected fuel
      | when transient fueling is disabled
  Fdes [g/s] : Inport
  Action Port : ActionPort  InitializeStates=reset
  Finj [g/s] : Outport
  wires:
  Fdes [g/s]/1 -> Finj [g/s]/1

== system motohawk_engine_lib/Model Fuel Puddle Mass/motohawk_TitleBlock ==

== system motohawk_engine_lib/Non-Linear Sensor Characterization (eqn)/If Action Subsystem ==
  In : Inport
  Action Port : ActionPort
  Out : Outport
  wires:
  In/1 -> Out/1

== system motohawk_engine_lib/Non-Linear Sensor Characterization (eqn)/If Action Subsystem2 ==
  In : Inport
  Action Port : ActionPort
  Out : Outport
  wires:
  In/1 -> Out/1

== system motohawk_engine_lib/Non-Linear Sensor Characterization (tbl)/If Action Subsystem ==
  In : Inport
  Action Port : ActionPort
  Out : Outport
  wires:
  In/1 -> Out/1

== system motohawk_engine_lib/Non-Linear Sensor Characterization (tbl)/If Action Subsystem1 ==
  In : Inport
  Action Port : ActionPort
  Out : Outport
  wires:
  In/1 -> Out/1

== system motohawk_engine_lib/Non-Linear Sensor Characterization (tbl)/If Action Subsystem2 ==
  In : Inport
  Action Port : ActionPort
  Out : Outport
  wires:
  In/1 -> Out/1

== system motohawk_engine_lib/Normalized Effective Combustion Chamber Temperature/CompareTo ==
  note: Check how input compares to 'val'
  In : Inport
  Constant : Constant  Value=val
  RelOp : RelationalOperator  Operator===  ZeroCross=off  InputSameDT=on
  Out : Outport
  wires:
  In/1 -> RelOp/1
  RelOp/1 -> Out/1
  Constant/1 -> RelOp/2

== system motohawk_engine_lib/Normalized Effective Combustion Chamber Temperature/Integrate an offset to ECT  Reset offset when engine is stopped. ==
  Integrand : Inport
  Reset : Inport  Port=2
  Enable : EnablePort
  Constant : Constant  Value=0
  Constant1 : Constant  Value=0
  Constant2 : Constant  Value=inf
  Integrator : Subsystem  mask(Discrete Integrator){samp_time=SampleTime}
      mask prompts: samp_time "Sample Time"
      mask help:
      | Resetable integrator with upper and lower windup limits.
      |
      | If 'Sample Time' is -1, then extra code and RAM will be generated to dynamically calculate dt.
      mask Display:
      | patch([0 0 1 1], 0.75*[0 0.075 0.075 0], [230/255 0/255 0/255])
      | patch([0 0 1 1], 0.75*[0.025 0.05 0.05 0.025], [150/255 0/255 0/255])
      | patch([0 0 1 1], 0.75*[0 0.025 0.025 0], [0/255 0/255 0/255])
      | 
      | disp('\fontsize{16}\bf\it\int dt', 'texmode', 'on')
  ECT Offset : Outport
  wires:
  Constant/1 -> Integrator/4(Min)
  Constant1/1 -> Integrator/3(IC)
  Integrand/1 -> Integrator/1(In)
  Integrator/1(Out) -> ECT Offset/1
  Reset/1 -> Integrator/2(Rst)
  Constant2/1 -> Integrator/5(Max)

== system motohawk_engine_lib/Normalized Effective Combustion Chamber Temperature/motohawk_TitleBlock ==
